simulink model "zad2model"  (R2012b)
settings: Solver=ode45  StartTime=0  StopTime=10.0  MinStep=0.1  RelTol=1e-10
libraries: simulink x1
settings Model: Creator=VoAnder  LastModifiedBy=VoAnder
settings SolverCC: InitialStep=0.1

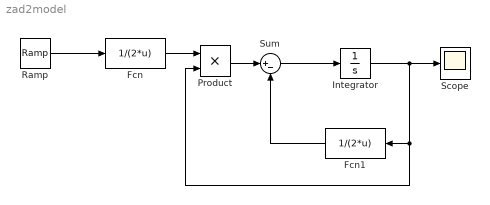
== system zad2model ==
  Fcn : Fcn  Expr=1/(2*u)
  Fcn1 : Fcn  Expr=1/(2*u)  SampleTime=1
  Integrator : Integrator  InitialCondition=0.1
  Product : Product  RndMeth=Zero
  Ramp : simulink/Sources/Ramp  slope=1  start=0  X0=0.1
  Scope : Scope
      settings: TimeRange=10
  Sum : Sum  Inputs=|+-
  wires:
  Ramp/1 -> Fcn/1
  Fcn/1 -> Product/1
  Product/1 -> Sum/1
  Sum/1 -> Integrator/1
  Fcn1/1 -> Sum/2
  Integrator/1 -> Product/2, Fcn1/1, Scope/1
